simulink model "simulation"  (R2016a)
settings: Solver=VariableStepAuto  StartTime=0.0  StopTime=10.0  RelTol=1e-3
libraries: aerolibatmos2 x2, aerolibasang x1
settings Model: Creator=Ian  LastModifiedBy=Ian
settings GRTTargetCC: GeneratePreprocessorConditionals=Use local settings

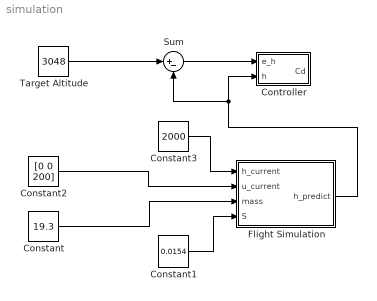
== system simulation ==
  Constant : Constant  Value=19.3
  Constant1 : Constant  Value=0.0154
  Constant2 : Constant  Value=[0 0 200]
  Constant3 : Constant  Value=2000
  Controller : Subsystem
  Flight Simulation : Subsystem
  Sum : Sum  Inputs=|+-
  Target Altitude : Constant  Value=3048
  wires:
  Sum/1 -> Controller/1("e_h ")
  Target Altitude/1 -> Sum/1
  Constant/1 -> Flight Simulation/3(mass)
  Constant1/1 -> Flight Simulation/4(S)
  Constant2/1 -> Flight Simulation/2(u_current)
  Constant3/1 -> Flight Simulation/1(h_current)
  Flight Simulation/1(h_predict) -> Sum/2, Controller/2(h)

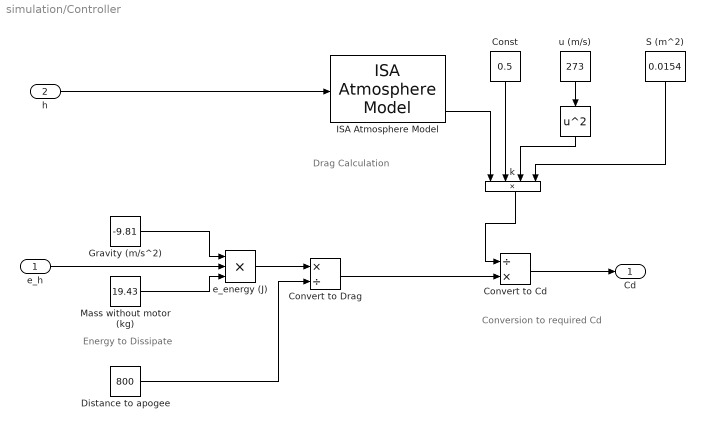
== system simulation/Controller ==
  note: Conversion to required Cd
  note: Energy to Dissipate
  note: Drag Calculation
  "e_h " : Inport
  h : Inport  Port=2
  " " : Math  Operator=square  SaturateOnIntegerOverflow=on
  Const : Constant  Value=0.5
  Convert to Cd : Product  Inputs=/*
  Convert to Drag : Product  Inputs=*/
  Distance to apogee : Constant  Value=800
  Gravity (m/s^2) : Constant  Value=-9.81
  ISA Atmosphere Model : aerolibatmos2/ISA Atmosphere Model  custom=off  g=9.80665  gamma=1.4  R=287.0531  L=0.0065  h_trop=11000  h_strat=20000  rho0=1.225  P0=101325  T0=288.15  h0=0
  Mass without motor (kg) : Constant  Value=19.43
  S (m^2) : Constant  Value=0.0154
  e_energy (J) : Product  Inputs=3
  k : Product  Inputs=4
  u (m/s) : Constant  Value=273
  Cd : Outport
  wires:
  Mass without motor (kg)/1 -> e_energy (J)/3
  "e_h "/1 -> e_energy (J)/2
  Gravity (m/s^2)/1 -> e_energy (J)/1
  Distance to apogee/1 -> Convert to Drag/2
  e_energy (J)/1 -> Convert to Drag/1
  u (m/s)/1 -> " "/1
  ISA Atmosphere Model/4 -> k/1
  " "/1 -> k/3
  S (m^2)/1 -> k/4
  Const/1 -> k/2
  Convert to Cd/1 -> Cd/1
  h/1 -> ISA Atmosphere Model/1
  k/1 -> Convert to Cd/1
  Convert to Drag/1 -> Convert to Cd/2

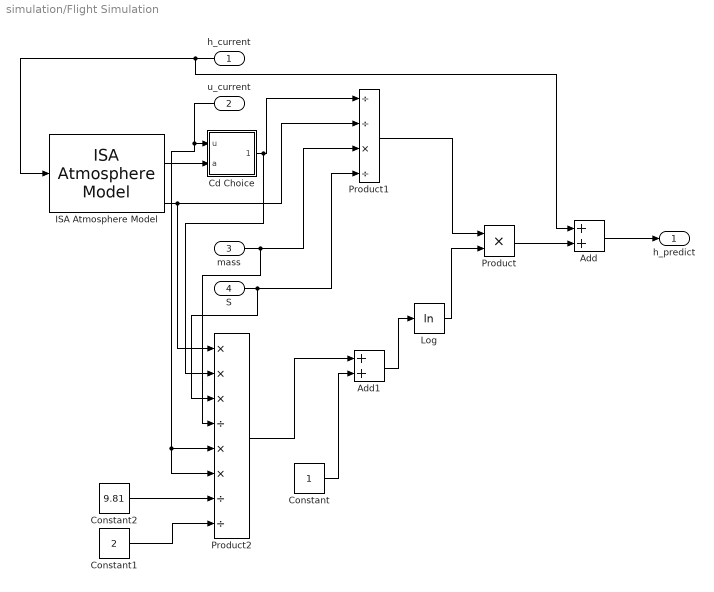
== system simulation/Flight Simulation ==
  h_current : Inport
  u_current : Inport  Port=2
  mass : Inport  Port=3
  S : Inport  Port=4
  " Log" : Math  Operator=log  SaturateOnIntegerOverflow=on
  Add : Sum
  Add1 : Sum
  Cd Choice : Subsystem
  Constant : Constant
  Constant1 : Constant  Value=2
  Constant2 : Constant  Value=9.81
  ISA Atmosphere Model : aerolibatmos2/ISA Atmosphere Model  custom=off  g=9.80665  gamma=1.4  R=287.0531  L=0.0065  h_trop=11000  h_strat=20000  rho0=1.225  P0=101325  T0=288.15  h0=0
  Product : Product
  Product1 : Product  Inputs=//*/
  Product2 : Product  Inputs=***/**//
  h_predict : Outport
  wires:
  h_current/1 -> Add/1, ISA Atmosphere Model/1
  ISA Atmosphere Model/2 -> Cd Choice/2(a)
  u_current/1 -> Product2/6, Product2/5, Cd Choice/1(u)
  Product/1 -> Add/2
  Cd Choice/1(Cdeff) -> Product2/2, Product1/1
  ISA Atmosphere Model/4 -> Product1/2, Product2/1
  mass/1 -> Product2/4, Product1/3
  S/1 -> Product2/3, Product1/4
  " Log"/1 -> Product/2
  Product1/1 -> Product/1
  Constant/1 -> Add1/2
  Add1/1 -> " Log"/1
  Constant1/1 -> Product2/8
  Constant2/1 -> Product2/7
  Product2/1 -> Add1/1
  Add/1 -> h_predict/1

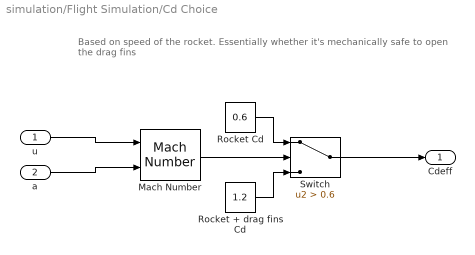
== system simulation/Flight Simulation/Cd Choice ==
  note: Based on speed of the rocket. Essentially whether it's mechanically safe
      | to open the drag fins
  u : Inport
  a : Inport  Port=2
  Mach Number : aerolibasang/Mach Number
  Rocket + drag fins Cd : Constant  Value=1.2
  Rocket Cd : Constant  Value=0.6
  Switch : Switch  Criteria=u2 > Threshold  Threshold=0.6
  Cdeff : Outport
  wires:
  Mach Number/1 -> Switch/2
  Rocket Cd/1 -> Switch/1
  Rocket + drag fins Cd/1 -> Switch/3
  u/1 -> Mach Number/1
  a/1 -> Mach Number/2
  Switch/1 -> Cdeff/1
